simulink model "useCaseMDL"  (R2024a)
settings: Solver=VariableStepAuto  StartTime=0.0  StopTime=10.0  RelTol=1e-3
undefined symbols (not defined in the file or in its folder): dem, gridLoc, originalReferencePath, res
libraries: roshelperlib x1, commrandsrc3 x1, dspstat3 x1
settings Model: Creator=cstabile  LastModifiedBy=cstabile
settings ConfigComp: CovAccelSimSupport=on

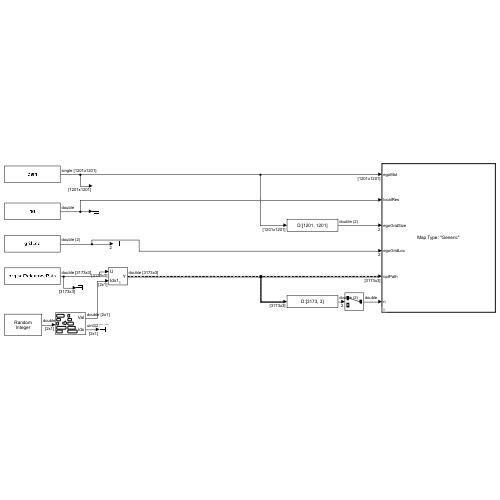
[thumbnail: Simulink's stored preview of the top-level diagram]
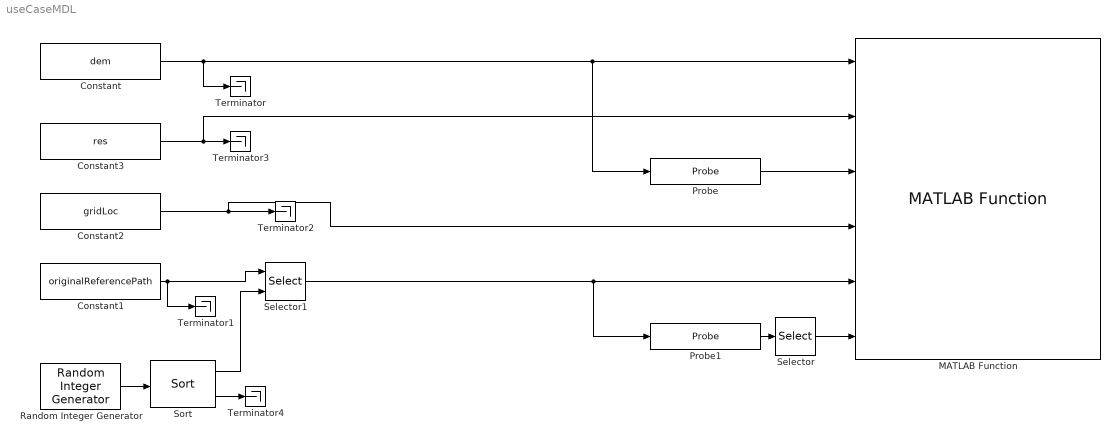
== system useCaseMDL ==
  Constant : Constant  Value=dem  VectorParams1D=off
  Constant1 : Constant  Value=originalReferencePath  VectorParams1D=off
  Constant2 : Constant  Value=gridLoc
  Constant3 : Constant  Value=res
  MATLAB Function : roshelperlib/MATLAB Function  mapType="\"Generic\""
  Probe : Probe  ProbeWidth=off  ProbeSampleTime=off  ProbeComplexSignal=off  ProbeSignalDimensions=on
  Probe1 : Probe  ProbeWidth=off  ProbeSampleTime=off  ProbeComplexSignal=off  ProbeSignalDimensions=on
  Random Integer Generator : commrandsrc3/Random Integer Generator  SetSize=3000  SeedSource=Auto  Seed=0  SampleTime=1  SamplesPerFrame=2  OutputDataType=double  SimulateUsing=Interpreted execution
  Selector : Selector  InputPortWidth=2  IndexOptions=Index vector (dialog)  Indices=1  OutputSizes=1
  Selector1 : Selector  NumberOfDimensions=2  InputPortWidth=3  IndexOptions=Starting and ending indices (port),Select all  Indices=[1 3],1  OutputSizes=1,1
  Sort : dspstat3/Sort  otype=Value and Index  dir=Ascending  sortAlg=Quick sort  roundingMode=Floor  overflowMode=off  accumDataTypeStr=Inherit: Same as product output  accumLastDataTypeStr=Inherit: Same as product output
  Terminator{,1..4} (5 alike) : Terminator
  wires:
  Constant1/1 -> Selector1/1, Terminator1/1
  Selector/1 -> MATLAB Function/6
  Probe1/1 -> Selector/1
  Constant3/1 -> MATLAB Function/2, Terminator3/1
  Constant/1 -> Probe/1, MATLAB Function/1, Terminator/1
  Constant2/1 -> MATLAB Function/4, Terminator2/1
  Probe/1 -> MATLAB Function/3
  Random Integer Generator/1 -> Sort/1
  Sort/1 -> Selector1/2
  Sort/2 -> Terminator4/1
  Selector1/1 -> Probe1/1, MATLAB Function/5
